simulink model "spot410_simOnboard"  (R2024b)
settings: Solver=ode4  StartTime=0.0  StopTime=tsim  FixedStep=baseRate  RelTol=1e-6  AbsTol=1e-6
values from neighbouring files (symbols this model uses):
  baseRate = paramEst(phase,coord).k2    [SpotEstimator.m]
undefined symbols (not defined in the file or in its folder): a1, a2, a3, b0, b1, b2, b3, dataRate, DiscIntNeverNeededParam, drop_states_ARM, drop_states_BLACK, drop_states_BLUE, drop_states_RED, F_black_X_nominal, F_black_Y_nominal, F_blue_X_nominal, F_blue_Y_nominal, F_red_X_nominal, F_red_Y_nominal, F_thrusters_BLACK, F_thrusters_BLUE, F_thrusters_RED, Gamma1_el, Gamma1_sh, Gamma1_wr, Gamma2_el, Gamma2_sh, Gamma2_wr, Gamma3_el, Gamma3_sh, Gamma3_wr, Gamma4_el, Gamma4_sh, Gamma4_wr, Gamma5_el, Gamma5_sh, Gamma5_wr, Gamma6_el, Gamma6_sh, Gamma6_wr, home_states_BLACK, home_states_BLUE, home_states_RED, IBLACK, IBLUE, IDIST, IEE, init_states_BLACK, init_states_BLUE, init_states_RED, IPROX, IRED, K_BLACK, K_BLUE, K_RED, Kd_elarm, Kd_sharm, Kd_tb, Kd_tblue, Kd_tr ... (+51)
libraries: simulink x30, nvidiaSharedBlocks x19, MainLibrary x5, dspinverses x3, nvidiaIMUSensorslib x1
(part 8 of 8)

== matlab function spot410_simOnboard/PhaseSpace Camera Code/Use Hardware to Obtain States/Receive and Process Phasespace Data/Check for Sychronization/MATLAB Function ==
  data: StartClock output; RedReceiving input; BlackReceiving input; BlueReceiving input; platformSelection parameter
function StartClock = CheckForSync(RedReceiving, BlackReceiving, BlueReceiving, platformSelection)
        
    StartClock = 0;
    
    if (platformSelection == 1)
        
        if RedReceiving == 1

            StartClock = 1;

        else

            StartClock = 0;

        end
        
    elseif (platformSelection == 2)
        
        if BlackReceiving == 1

            StartClock = 1;

        else

            StartClock = 0;

        end  
        
    elseif (platformSelection == 3)
        
        if RedReceiving == 1 && BlackReceiving == 1

            StartClock = 1;

        else

            StartClock = 0;

        end    
        
    elseif (platformSelection == 4)
        
        if RedReceiving == 1 && BlackReceiving == 1

            StartClock = 1;

        else

            StartClock = 0;

        end
        
    elseif (platformSelection == 5)
        
        if RedReceiving == 1

            StartClock = 1;

        else

            StartClock = 0;

        end
        
    elseif (platformSelection == 6)
        
        if BlueReceiving == 1

            StartClock = 1;

        else

            StartClock = 0;

        end
        
    elseif (platformSelection == 7)
        
        if RedReceiving == 1 && BlueReceiving == 1

            StartClock = 1;

        else

            StartClock = 0;

        end
        
    elseif (platformSelection == 8)
        
        if RedReceiving == 1 && BlackReceiving == 1 && BlueReceiving == 1

            StartClock = 1;

        else

            StartClock = 0;

        end
        
    elseif (platformSelection == 9)
        
        if BlackReceiving == 1 && BlueReceiving == 1

            StartClock = 1;

        else

            StartClock = 0;

        end
                           
    elseif (platformSelection == 10)
        
        if RedReceiving == 1 && BlueReceiving == 1

            StartClock = 1;

        else

            StartClock = 0;

        end
        
    elseif (platformSelection == 11)
        
        if RedReceiving == 1 && BlackReceiving == 1 && BlueReceiving == 1

            StartClock = 1;

        else

            StartClock = 0;

        end
        
    end



end

== matlab function spot410_simOnboard/3 - Control/Default LQR Control (RED)/Calculate Error/MATLAB Function ==
  data: Rz_path input; Rz_error output; Rz_measured input
function Rz_error = SmoothAngularDifference(Rz_path, Rz_measured)

    Rz_error = mod(Rz_measured-Rz_path+pi, 2*pi)-pi;


end

== matlab function spot410_simOnboard/3 - Control/Default LQR Control (BLACK)/Calculate Error/MATLAB Function ==
  data: Rz_path input; Rz_error output; Rz_measured input
function Rz_error = SmoothAngularDifference(Rz_path, Rz_measured)

    Rz_error = mod(Rz_measured-Rz_path+pi, 2*pi)-pi;


end

== matlab function spot410_simOnboard/3 - Control/Default PD Control (RED)/Calculate Error/MATLAB Function ==
  data: Rz_path input; Rz_error output; Rz_measured input
function Rz_error = SmoothAngularDifference(Rz_path, Rz_measured)

    Rz_error = mod(Rz_measured-Rz_path+pi, 2*pi)-pi;


end
